simulink subsystem "pololu_37D_hardware_interface"  (R2023b)
settings: Solver=VariableStepAuto  StartTime=0.0  StopTime=10.0  RelTol=1e-3
model mask{Ts=0.005, pwmFreq=2000}
  mask prompts: Ts "Sampling Time"; pwmFreq "PWM Frequency"
libraries: mbedblockslib x3, stm_qeplib x1
settings Model: Creator=kiraa  LastModifiedBy=kiraa

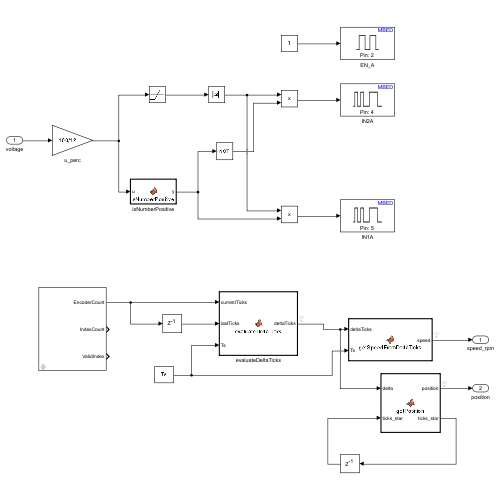
[thumbnail: Simulink's stored preview of the top-level diagram]
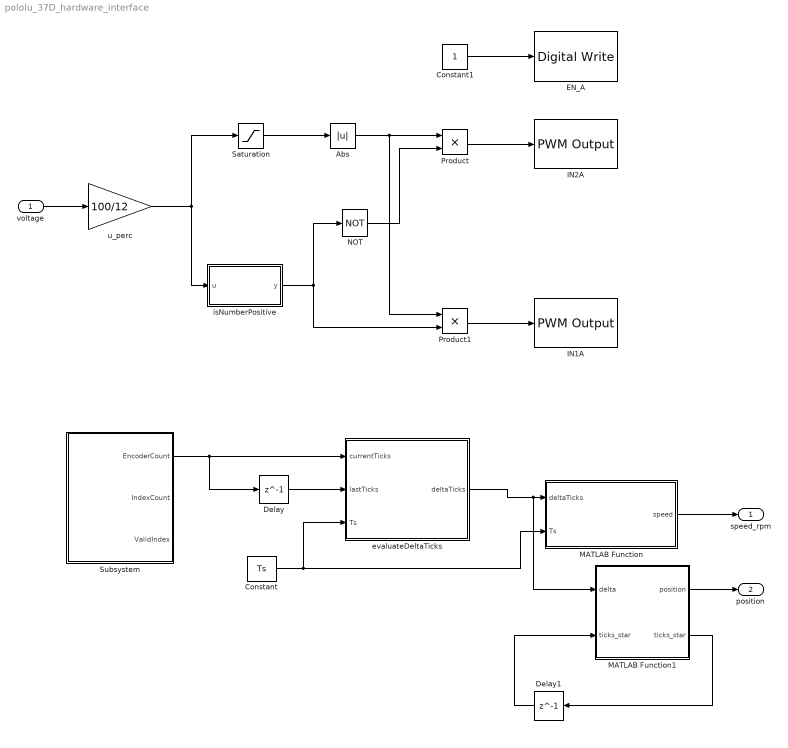
== system pololu_37D_hardware_interface ==
  voltage : Inport
  Abs : Abs  SaturateOnIntegerOverflow=off
  Constant : Constant  Value=Ts
  Constant1 : Constant
  Delay : Delay  DelayLength=1
  Delay1 : Delay  DelayLength=1
  EN_A : mbedblockslib/Digital Write  Pin=2  Direction=output
      settings: LibrarySourceBlock=stmnucleorootlib/Common/Digital Write
  IN1A : mbedblockslib/PWM Output  Pin=5  EnableInputFrequency=off  InitialFrequency=pwmFreq  InitialDutyCycle=50  NotificationType=None
      settings: LibrarySourceBlock=stmnucleorootlib/Common/PWM Output
  IN2A : mbedblockslib/PWM Output  Pin=4  EnableInputFrequency=off  InitialFrequency=pwmFreq  InitialDutyCycle=50  NotificationType=None
      settings: LibrarySourceBlock=stmnucleorootlib/Common/PWM Output
  MATLAB Function : MATLAB Function  TreatAsAtomicUnit=on
  MATLAB Function1 : MATLAB Function  TreatAsAtomicUnit=on
  NOT : Logic  Operator=NOT  AllPortsSameDT=off  OutDataTypeStr=boolean
  Product : Product
  Product1 : Product
  Saturation : Saturate  UpperLimit=100  LowerLimit=-100
  Subsystem : Subsystem  mask{Ts=Ts}
      mask prompts: Ts "Sampling Time"
  evaluateDeltaTicks : MATLAB Function  TreatAsAtomicUnit=on
  isNumberPositive : MATLAB Function  TreatAsAtomicUnit=on
  u_perc : Gain  Gain=100/12
  speed_rpm : Outport
  position : Outport  Port=2
  wires:
  Delay1/1 -> MATLAB Function1/2("ticks_star ")
  evaluateDeltaTicks/1(deltaTicks) -> MATLAB Function1/1(delta), MATLAB Function/1(deltaTicks)
  MATLAB Function1/2(ticks_star) -> Delay1/1
  Subsystem/1(EncoderCount) -> Delay/1, evaluateDeltaTicks/1(currentTicks)
  Delay/1 -> evaluateDeltaTicks/2(lastTicks)
  Constant/1 -> MATLAB Function/2(Ts), evaluateDeltaTicks/3(Ts)
  MATLAB Function/1(speed) -> speed_rpm/1
  MATLAB Function1/1(position) -> position/1
  Constant1/1 -> EN_A/1
  Saturation/1 -> Abs/1
  isNumberPositive/1(y) -> Product1/2, NOT/1
  Product1/1 -> IN1A/1
  u_perc/1 -> Saturation/1, isNumberPositive/1(u)
  NOT/1 -> Product/2
  Product/1 -> IN2A/1
  Abs/1 -> Product1/1, Product/1
  voltage/1 -> u_perc/1

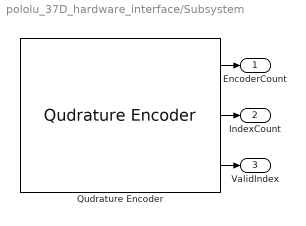
== system pololu_37D_hardware_interface/Subsystem ==
  Qudrature Encoder : stm_qeplib/Qudrature Encoder  SampleTime=Ts
  EncoderCount : Outport
  IndexCount : Outport  Port=2
  ValidIndex : Outport  Port=3
  wires:
  Qudrature Encoder/1 -> EncoderCount/1
  Qudrature Encoder/3 -> ValidIndex/1
  Qudrature Encoder/2 -> IndexCount/1

== matlab function pololu_37D_hardware_interface/isNumberPositive ==
  data: u input; y output
function y = isNumberPositive(u)
if u>0
    y = 1;
else
    y = 0;
end

== matlab function pololu_37D_hardware_interface/MATLAB Function ==
  data: deltaTicks input; speed output; Ts input
function speed = getSpeedFromDeltaTicks(deltaTicks,Ts)
    speed = deltaTicks * 60 /(8400*Ts);
end

== matlab function pololu_37D_hardware_interface/MATLAB Function1 ==
  data: delta input; position output; ticks_star input; ticks_star output
function [position, ticks_star] = getPosition(delta, ticks_star)
    ticks_star = double(ticks_star+delta);
    completeTheta = 2*pi*ticks_star/(8400); %ogni 8400 ho un numero intero di angoli giro
    position = sign(completeTheta)*mod(abs(completeTheta),2*pi);
end

== matlab function pololu_37D_hardware_interface/evaluateDeltaTicks ==
  data: currentTicks input; deltaTicks output; lastTicks input; Ts input
function deltaTicks = evaluateDeltaTicks(currentTicks, lastTicks, Ts)

currentTicks = double(currentTicks);
lastTicks = double(lastTicks);

if abs(currentTicks-lastTicks) <= ceil(12600*Ts)
    deltaTicks = currentTicks-lastTicks;
else
    if lastTicks>currentTicks
        deltaTicks = currentTicks-lastTicks+2^16-1;
    else
        deltaTicks = currentTicks-lastTicks-(2^16-1);
    end
end
